simulink model "FOC_basic4_CurrentCtrl_SVPWM"  (R2020b)
settings: Solver=FixedStepAuto  StartTime=0.0  StopTime=1  FixedStep=Ts  MaxStep=0.0005  RelTol=1e-3
InitFcn:
  | FOC;
undefined symbols (not defined in the file): innerPI, motor
libraries: mcbcontrolslib x2, pid_lib x2, mcbplantlib x1, autolibpmsminterior x1
settings Model: Creator=k  LastModifiedBy=k

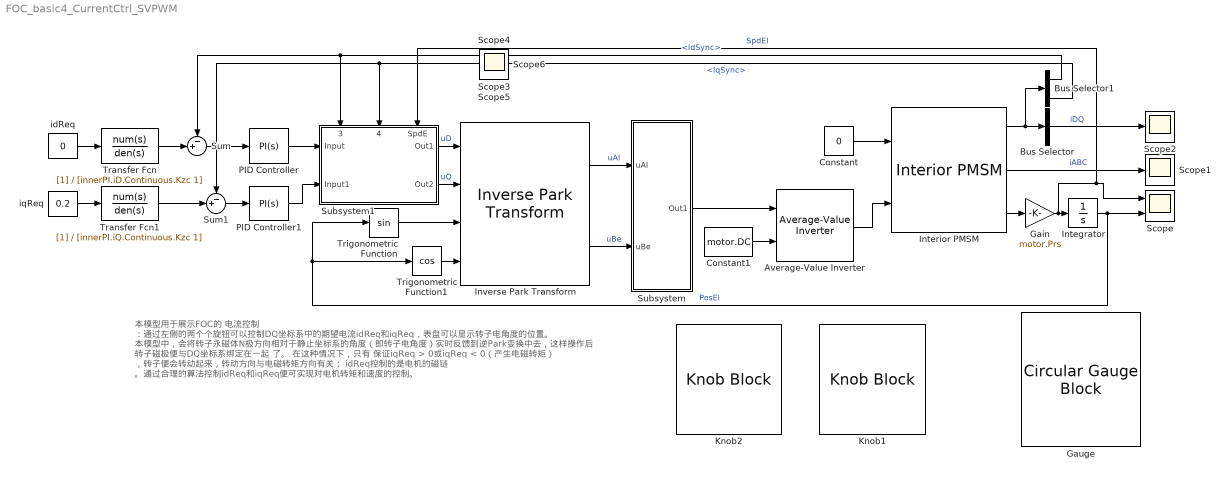
== system FOC_basic4_CurrentCtrl_SVPWM ==
  note: 本模型用于展示FOC的 电流控制 ：通过左侧的两个个旋钮可以控制DQ坐标系中的期望电流idReq和iqReq，表盘可以显示转子电角度的位置。
      |
      | 本模型中，会将转子永磁体N极方向相对于静止坐标系的角度（即转子电角度）实时反馈到逆Park变换中去，这样操作后 转子磁极便与DQ坐标系绑定在一起 了。
      |
      | 在这种情况下，只有 保证iqReq > 0或iqReq < 0（产生电磁转矩） ，转子便会转动起来，转动方向与电磁转矩方向有关； idReq控制的是电机的磁链 。通过合理的算法控制idReq和iqReq便可实现对电机转矩和速度的控制。
  Average-Value Inverter : mcbplantlib/Average-Value Inverter
  Bus Selector : BusSelector  OutputSignals=IdSync,IqSync  OutputAsBus=on
  Bus Selector1 : BusSelector  OutputSignals=IdSync,IqSync
  Constant : Constant  Value=0
  Constant1 : Constant  Value=motor.DC
  Gain : Gain  Gain=motor.Prs
  Gauge : CircularGaugeBlock  ScaleMin=-3.14  ScaleMax=3.14  TickInterval=1.57
  Integrator : Integrator  WrapState=on
  Interior PMSM : autolibpmsminterior/Interior PMSM  port_config=Torque  sim_type=Continuous  Ts=0.001  P=motor.Prs  Rs=motor.Rs  Ldq=[motor.Ld motor.Lq]  KConstText=Permanent flux linkage constant (lambda_pm):  lambda_pm=motor.Flux  Ke=159.9771  mechanical=[motor.J, motor.B, motor.Tf]  idq0=[0 0]  theta_init=0  omega_init=0  KConst=motor.Flux  lambda_pm_calc=motor.Flux  Kt=0.07  RefBlkName='autolibpmsminterior/Interior PMSM'  aMode=5
      settings: SourceProductBaseCode=PW,MT,UV,VE,VP
  Inverse Park Transform : mcbcontrolslib/Inverse Park Transform  AxisAlignment=D-axis
  Knob1 : KnobBlock  ScaleMin=-1  ScaleMax=1
  Knob2 : KnobBlock  ScaleMin=-1  ScaleMax=1
  PID Controller : pid_lib/PID Controller  Controller=PI  Form=Parallel  TimeDomain=Continuous-time  UseExternalTs=off  SampleTime=-1  IntegratorMethod=Forward Euler  FilterMethod=Forward Euler  ControllerParametersSource=internal  P=innerPI.iD.Continuous.Kp  I=innerPI.iD.Continuous.Ki  D=0  UseFilter=on  N=100  TunerSelectOption=Transfer Function Based (PID Tuner App)  InitialConditionSource=internal  InitialConditionForIntegrator=0  InitialConditionForFilter=0  DifferentiatorICPrevScaledInput=0  ExternalReset=none  TrackingMode=off  Kt=1  LimitOutput=off  SatLimitsSource=internal  UpperSaturationLimit=inf  LowerSaturationLimit=-inf  LinearizeAsGain=on  AntiWindupMode=none  Kb=1  POutMin=[]  POutMax=[]  IOutMin=[]  IOutMax=[]  DOutMin=[]  DOutMax=[]  NOutMin=[]  NOutMax=[]  SumOutMin=[]  SumOutMax=[]  SaturationOutMin=[]  SaturationOutMax=[]  PParamMin=[]  PParamMax=[]  IParamMin=[]  IParamMax=[]  DParamMin=[]  DParamMax=[]  NParamMin=[]  NParamMax=[]  KbParamMin=[]  KbParamMax=[]  KtParamMin=[]  KtParamMax=[]  KbOutMin=[]  KbOutMax=[]  KtOutMin=[]  KtOutMax=[]  IntegratorOutMin=[]  IntegratorOutMax=[]  FilterOutMin=[]  FilterOutMax=[]  SumI1OutMin=[]  SumI1OutMax=[]  SumI2OutMin=[]  SumI2OutMax=[]  SumI3OutMin=[]  SumI3OutMax=[]  SumI4OutMin=[]  SumI4OutMax=[]  SumDOutMin=[]  SumDOutMax=[]  DifferentiatorOutMin=[]  DifferentiatorOutMax=[]  FilterDiffOutCoefMin=[]  FilterDiffOutCoefMax=[]  ReciprocalOutMin=[]  ReciprocalOutMax=[]  SumDenOutMin=[]  SumDenOutMax=[]  SumNumOutMin=[]  SumNumOutMax=[]  DivideOutMin=[]  DivideOutMax=[]  UdiffTsProdOutMin=[]  UdiffTsProdOutMax=[]  NTsProdOutMin=[]  NTsProdOutMax=[]  UintegralTsProdOutMin=[]  UintegralTsProdOutMax=[]  UngainTsProdOutMin=[]  UngainTsProdOutMax=[]  IntegratorContinuousStateAttributes=''  IntegratorStateMustResolveToSignalObject=off  IntegratorRTWStateStorageClass=Auto  FilterContinuousStateAttributes=''  FilterStateMustResolveToSignalObject=off  FilterRTWStateStorageClass=Auto  ParallelPVariant=InternalParameters  IdealPVariant=Disabled  IVariant=InternalParameters  DVariant=Disabled  IntegratorVariant=Continuous  SatVariant=Disabled  AWVariant=Passthrough  PCopyVariant=Disabled  TRVariant=Disabled  FdbkBlocksVariant=Forward  IdealPFdbkVariant=Disabled  SatFdbkVariant=Disabled  DerivativeFilterVariant=Disabled  NVariant=Disabled  NCopyVariant=Disabled_SignalSpec  FilterICVariant=Disabled  IntegratorICVariant=InternalICs  ExternalResetVariant=Disabled  TRSumVariant=Passthrough  SumFdbkVariant=Disabled  SumVariant=Sum_PI  TsampFilterVariant=InternalTs  TsampNgainVariant=Passthrough  TsampIntegralVariant=Passthrough  ExternalSaturationOutDataTypeStr=Inherit: Same as second input
  PID Controller1 : pid_lib/PID Controller  Controller=PI  Form=Parallel  TimeDomain=Continuous-time  UseExternalTs=off  SampleTime=-1  IntegratorMethod=Forward Euler  FilterMethod=Forward Euler  ControllerParametersSource=internal  P=innerPI.iQ.Continuous.Kp  I=innerPI.iQ.Continuous.Ki  D=0  UseFilter=on  N=100  TunerSelectOption=Transfer Function Based (PID Tuner App)  InitialConditionSource=internal  InitialConditionForIntegrator=0  InitialConditionForFilter=0  DifferentiatorICPrevScaledInput=0  ExternalReset=none  TrackingMode=off  Kt=1  LimitOutput=off  SatLimitsSource=internal  UpperSaturationLimit=inf  LowerSaturationLimit=-inf  LinearizeAsGain=on  AntiWindupMode=none  Kb=1  POutMin=[]  POutMax=[]  IOutMin=[]  IOutMax=[]  DOutMin=[]  DOutMax=[]  NOutMin=[]  NOutMax=[]  SumOutMin=[]  SumOutMax=[]  SaturationOutMin=[]  SaturationOutMax=[]  PParamMin=[]  PParamMax=[]  IParamMin=[]  IParamMax=[]  DParamMin=[]  DParamMax=[]  NParamMin=[]  NParamMax=[]  KbParamMin=[]  KbParamMax=[]  KtParamMin=[]  KtParamMax=[]  KbOutMin=[]  KbOutMax=[]  KtOutMin=[]  KtOutMax=[]  IntegratorOutMin=[]  IntegratorOutMax=[]  FilterOutMin=[]  FilterOutMax=[]  SumI1OutMin=[]  SumI1OutMax=[]  SumI2OutMin=[]  SumI2OutMax=[]  SumI3OutMin=[]  SumI3OutMax=[]  SumI4OutMin=[]  SumI4OutMax=[]  SumDOutMin=[]  SumDOutMax=[]  DifferentiatorOutMin=[]  DifferentiatorOutMax=[]  FilterDiffOutCoefMin=[]  FilterDiffOutCoefMax=[]  ReciprocalOutMin=[]  ReciprocalOutMax=[]  SumDenOutMin=[]  SumDenOutMax=[]  SumNumOutMin=[]  SumNumOutMax=[]  DivideOutMin=[]  DivideOutMax=[]  UdiffTsProdOutMin=[]  UdiffTsProdOutMax=[]  NTsProdOutMin=[]  NTsProdOutMax=[]  UintegralTsProdOutMin=[]  UintegralTsProdOutMax=[]  UngainTsProdOutMin=[]  UngainTsProdOutMax=[]  IntegratorContinuousStateAttributes=''  IntegratorStateMustResolveToSignalObject=off  IntegratorRTWStateStorageClass=Auto  FilterContinuousStateAttributes=''  FilterStateMustResolveToSignalObject=off  FilterRTWStateStorageClass=Auto  ParallelPVariant=InternalParameters  IdealPVariant=Disabled  IVariant=InternalParameters  DVariant=Disabled  IntegratorVariant=Continuous  SatVariant=Disabled  AWVariant=Passthrough  PCopyVariant=Disabled  TRVariant=Disabled  FdbkBlocksVariant=Forward  IdealPFdbkVariant=Disabled  SatFdbkVariant=Disabled  DerivativeFilterVariant=Disabled  NVariant=Disabled  NCopyVariant=Disabled_SignalSpec  FilterICVariant=Disabled  IntegratorICVariant=InternalICs  ExternalResetVariant=Disabled  TRSumVariant=Passthrough  SumFdbkVariant=Disabled  SumVariant=Sum_PI  TsampFilterVariant=InternalTs  TsampNgainVariant=Passthrough  TsampIntegralVariant=Passthrough  ExternalSaturationOutDataTypeStr=Inherit: Same as second input
  Scope : Scope  NumInputPorts=2
  Scope{1..6} (6 alike) : Scope
  Subsystem : Subsystem
  Subsystem1 : Subsystem
      settings: PortSchema="{\"entries\":[{\"content\":{\"sides\":[{\"content\":{\"connectorIds\":[\"In1\",\"In2\"]},\"type\":\"ConnectorPlacement.EquallySpacedRectSide\",\"uuid\":\"da513fce-1bba-488f-9066-1c6e94016250\"},{\"content\":{\"connectorIds\":[\"Out1\",\"Out2\"],\"side\":\"RIGHT\"},\"type\":\"ConnectorPlacement.EquallySpacedRectSide\",\"uuid\":\"eadffa07-b25a-47cd-9c66-7794e561c7b0\"},{\"content\":{\"connectorIds\":[\"In3\",\"In4\",\"In5\"],\"side\":\"TOP\"},\"type\":\"ConnectorPlacement.EquallySpacedRectSide\",\"uuid\":\"6a54559a-6875-4e90-8096-133911583f85\"},{\"content\":{\"connectorIds\":[],\"side\":\"HIDDEN\"},\"type\":\"ConnectorPlacement.EquallySpacedRectSide\",\"uuid\":\"5dce9a10-9026-4f74-b8b5-e91710980954\"}]},\"type\":\"ConnectorPlacement.EquallySpacedConnector\",\"uuid\":\"af0a4674-08b6-4fea-be1c-7d21f073a6e8\"}],\"packageUris\":[\"http://schema.mathworks.com/mf0/Connector/R2020b\"],\"version\":\"1.0\"}"
      mask Display: disp('Decouple');
  Sum : Sum  Inputs=-+|
  Sum1 : Sum  Inputs=-+|
  Transfer Fcn : TransferFcn  Denominator=[innerPI.iD.Continuous.Kzc 1]
  Transfer Fcn1 : TransferFcn  Denominator=[innerPI.iQ.Continuous.Kzc 1]
  Trigonometric Function : Trigonometry
  Trigonometric Function1 : Trigonometry  Operator=cos
  idReq : Constant  Value=0
  iqReq : Constant  Value=0.2
  wires:
  Interior PMSM/3 -> Gain/1
  Interior PMSM/2 -> Scope1/1  "iABC"
  Interior PMSM/1 -> Bus Selector1/1, Bus Selector/1
  Bus Selector/1 -> Scope2/1  "iDQ"
  Gain/1 -> Scope/1, Subsystem1/5(SpdE), Integrator/1  "SpdEl"
  idReq/1 -> Transfer Fcn/1
  Sum/1 -> PID Controller/1
  Bus Selector1/1 -> Subsystem1/3(<IdSync>), Sum/1  "<IdSync>"
  iqReq/1 -> Transfer Fcn1/1
  Sum1/1 -> PID Controller1/1
  Bus Selector1/2 -> Subsystem1/4(<IqSync>), Sum1/1  "<IqSync>"
  PID Controller/1 -> Subsystem1/1(Input)
  PID Controller1/1 -> Subsystem1/2(Input1)
  Subsystem1/1(Out1) -> Inverse Park Transform/1  "uD"
  Subsystem1/2(Out2) -> Inverse Park Transform/2  "uQ"
  Transfer Fcn/1 -> Sum/2
  Transfer Fcn1/1 -> Sum1/2
  Constant/1 -> Interior PMSM/1
  Integrator/1 -> Trigonometric Function1/1, Trigonometric Function/1, Scope/2  "PosEl"
  Trigonometric Function1/1 -> Inverse Park Transform/4
  Trigonometric Function/1 -> Inverse Park Transform/3
  Constant1/1 -> Average-Value Inverter/2
  Average-Value Inverter/1 -> Interior PMSM/2
  Inverse Park Transform/1 -> Subsystem/1(uAl)  "uAl"
  Inverse Park Transform/2 -> Subsystem/2(uBe)  "uBe"
  Subsystem/1(Out1) -> Average-Value Inverter/1

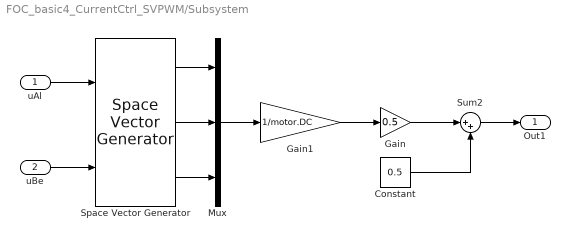
== system FOC_basic4_CurrentCtrl_SVPWM/Subsystem ==
  uAl : Inport
  uBe : Inport  Port=2
  Constant : Constant  Value=0.5
  Gain : Gain  Gain=0.5
  Gain1 : Gain  Gain=1/motor.DC
  Mux : Mux  Inputs=3
  Space Vector Generator : mcbcontrolslib/Space Vector Generator
      settings: SourceProductBaseCode=MT
  Sum2 : Sum  Inputs=|++
  Out1 : Outport
  wires:
  uBe/1 -> Space Vector Generator/2
  Space Vector Generator/2 -> Mux/2
  Space Vector Generator/1 -> Mux/1
  Space Vector Generator/3 -> Mux/3
  uAl/1 -> Space Vector Generator/1
  Mux/1 -> Gain1/1
  Constant/1 -> Sum2/2
  Gain/1 -> Sum2/1
  Sum2/1 -> Out1/1
  Gain1/1 -> Gain/1

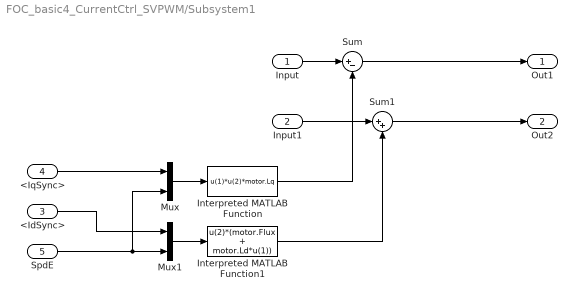
== system FOC_basic4_CurrentCtrl_SVPWM/Subsystem1 ==
  Input : Inport
  Input1 : Inport  Port=2
  <IdSync> : Inport  Port=3
  <IqSync> : Inport  Port=4
  SpdE : Inport  Port=5
  Interpreted MATLAB Function : MATLABFcn  MATLABFcn=u(1)*u(2)*motor.Lq
  Interpreted MATLAB Function1 : MATLABFcn  MATLABFcn=u(2)*(motor.Flux + motor.Ld*u(1))
  Mux : Mux  Inputs=2
  Mux1 : Mux  Inputs=2
  Sum : Sum  Inputs=|+-
  Sum1 : Sum  Inputs=|++
  Out1 : Outport
  Out2 : Outport  Port=2
  wires:
  SpdE/1 -> Mux/2, Mux1/2
  Mux/1 -> Interpreted MATLAB Function/1
  Mux1/1 -> Interpreted MATLAB Function1/1
  <IqSync>/1 -> Mux/1
  <IdSync>/1 -> Mux1/1
  Input/1 -> Sum/1
  Input1/1 -> Sum1/1
  Interpreted MATLAB Function/1 -> Sum/2
  Interpreted MATLAB Function1/1 -> Sum1/2
  Sum/1 -> Out1/1
  Sum1/1 -> Out2/1
